simulink model "TestGuiSetpointHandler"  (R2016b)
settings: Solver=FixedStepAuto  StartTime=0.0  StopTime=inf  FixedStep=0.002  RelTol=1e-3  EnableMultiTasking=on
libraries: slrtlib x2
settings Model: SimulationMode=external  Creator=march  LastModifiedBy=march
settings SolverCC: EnableConcurrentExecution=on
settings DataIOCC: SaveFormat=StructureWithTime
settings OptimizationCC: BlockReduction=off  OptimizeBlockIOStorage=off  BufferReuse=off  GlobalBufferReuse=off  ExpressionFolding=off  LocalBlockOutputs=off
settings HardwareCC: ProdBitPerPointer=32  ProdBitPerSizeT=32  ProdBitPerPtrDiffT=32  ProdLargestAtomicFloat=None  ProdWordSize=32  ProdLongLongMode=on  ProdHWDeviceType=Generic->32-bit x86 compatible
settings RTWCC: SystemTargetFile=slrt.tlc  TemplateMakefile=slrt_default_tmf  Description=Simulink Real-Time  RTWCompilerOptimization=on

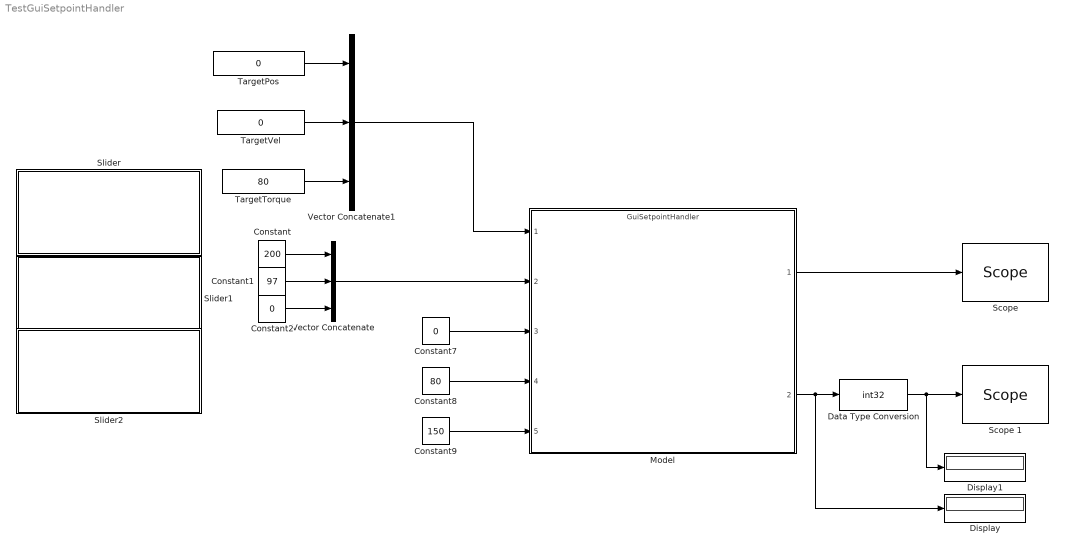
== system TestGuiSetpointHandler ==
  Constant : Constant  Value=200
  Constant1 : Constant  Value=97
  Constant2 : Constant  Value=0
  Constant7 : Constant  Value=0
  Constant8 : Constant  Value=80
  Constant9 : Constant  Value=150
  Data Type Conversion : DataTypeConversion  OutDataTypeStr=int32
  Display : Display
  Display1 : Display
  Model : ModelReference  ModelNameDialog=GuiSetpointHandler  SimulationMode=Normal  ModelReferenceVersion=1.22
  "Scope " : slrtlib/Displays and Logging/Scope   scopeno=1  scopetype=Target  autostart=on  viewmode=Graphical sliding  formatstr='%15.6f'  grid=on  ylimits=[-200,200]  nosamples=2500  noprepostsamples=0  interleave=1  triggermode=FreeRun  triggersignal=1  trigsignalfromport=off  triggerlevel=0.0  triggerslope=Either  triggerscope=1  triggersample=0  filename=data.dat  mode=Lazy  writesize=512  autorestart=off  dynamicfilemode=off  maxwritefilesize=512*1024^2
  Scope 1 : slrtlib/Displays and Logging/Scope   scopeno=2  scopetype=Target  autostart=on  viewmode=Numerical  formatstr='%15.6f'  grid=on  ylimits=[0,0]  nosamples=250  noprepostsamples=0  interleave=1  triggermode=FreeRun  triggersignal=1  trigsignalfromport=off  triggerlevel=0.0  triggerslope=Either  triggerscope=1  triggersample=0  filename=data.dat  mode=Lazy  writesize=512  autorestart=off  dynamicfilemode=off  maxwritefilesize=512*1024^2
  Slider : Subsystem  DialogController=hmiCreateDDGDialog  IsWebBlock=on  mask(MWDashboardBlock){webBlockId=74a66a5a-4541-4654-a565-17f35d4b1935, webBlockType=slider, ShowInLibBrowser=on, ShowInitialText=on, HMISrcModelName=TestGuiSetpointHandler}
      mask prompts: webBlockId "WebBlock Id"; webBlockType "WebBlock Type"; HMISrcModelName "Source Model"
      mask help: SimulinkHMI:dialogs:SliderDialogDesc
      mask Help: helpview([docroot '/mapfiles/simulink.map'], 'hmi_slider')
      mask Display:
      | if strcmp(get_param(bdroot(gcb),'BlockDiagramType'), 'library')
      |     image([(matlabroot) '/toolbox/simulink/hmi/icons/Slider.png']);
      | end
  Slider1 : Subsystem  DialogController=hmiCreateDDGDialog  IsWebBlock=on  mask(MWDashboardBlock){webBlockId=3f26eca4-6975-4227-bb64-2fe27ec89b6e, webBlockType=slider, ShowInLibBrowser=on, ShowInitialText=on, HMISrcModelName=TestGuiSetpointHandler}
      mask prompts: webBlockId "WebBlock Id"; webBlockType "WebBlock Type"; HMISrcModelName "Source Model"
      mask help: SimulinkHMI:dialogs:SliderDialogDesc
      mask Help: helpview([docroot '/mapfiles/simulink.map'], 'hmi_slider')
      mask Display:
      | if strcmp(get_param(bdroot(gcb),'BlockDiagramType'), 'library')
      |     image([(matlabroot) '/toolbox/simulink/hmi/icons/Slider.png']);
      | end
  Slider2 : Subsystem  DialogController=hmiCreateDDGDialog  IsWebBlock=on  mask(MWDashboardBlock){webBlockId=3df49d9d-fcd5-4737-ac0a-669262cebfea, webBlockType=slider, ShowInLibBrowser=on, ShowInitialText=on, HMISrcModelName=TestGuiSetpointHandler}
      mask prompts: webBlockId "WebBlock Id"; webBlockType "WebBlock Type"; HMISrcModelName "Source Model"
      mask help: SimulinkHMI:dialogs:SliderDialogDesc
      mask Help: helpview([docroot '/mapfiles/simulink.map'], 'hmi_slider')
      mask Display:
      | if strcmp(get_param(bdroot(gcb),'BlockDiagramType'), 'library')
      |     image([(matlabroot) '/toolbox/simulink/hmi/icons/Slider.png']);
      | end
  TargetPos : Constant  Value=0
  TargetTorque : Constant  Value=80
  TargetVel : Constant  Value=0
  Vector Concatenate : Concatenate  NumInputs=3
  Vector Concatenate1 : Concatenate  NumInputs=3
  wires:
  Constant1/1 -> Vector Concatenate/2
  Constant/1 -> Vector Concatenate/1
  Constant2/1 -> Vector Concatenate/3
  Vector Concatenate/1 -> Model/2
  Vector Concatenate1/1 -> Model/1
  Constant7/1 -> Model/3
  Constant9/1 -> Model/5
  Constant8/1 -> Model/4
  Model/1 -> "Scope "/1
  Model/2 -> Display/1, Data Type Conversion/1
  Data Type Conversion/1 -> Display1/1, Scope 1/1
  TargetVel/1 -> Vector Concatenate1/2
  TargetPos/1 -> Vector Concatenate1/1
  TargetTorque/1 -> Vector Concatenate1/3

== system TestGuiSetpointHandler/Slider ==

== system TestGuiSetpointHandler/Slider1 ==

== system TestGuiSetpointHandler/Slider2 ==
